simulink model "c28x_i2c_sensor"  (R2023b)
settings: Solver=FixedStepDiscrete  StartTime=0.0  StopTime=Inf  FixedStep=Auto  RelTol=1e-3  EnableMultiTasking=on
undefined symbols (not defined in the file): dataType
libraries: c280xlib x7, simulink x3, demo_controls x1, svdschedulerlib x1, svdutilitieslib x1
settings Model: SimulationMode=external  ExtModeTrigDuration=8  Creator=The MathWorks, Inc.  LastModifiedBy=13571
settings SolverCC: AlgebraicLoopSolver=TrustRegion  AutoInsertRateTranBlk=on
settings DataIOCC: LimitDataPoints=on  SaveFormat=Array  SaveOutput=off  SaveTime=off  ReturnWorkspaceOutputs=off
settings OptimizationCC: BlockReduction=off  ConditionallyExecuteInputs=off  DefaultParameterBehavior=Inlined  DefaultUnderspecifiedDataType=single  OptimizeBlockIOStorage=off  BufferReuse=off  GlobalBufferReuse=off  ExpressionFolding=off  ExpressionDepthLimit=2147483647  LocalBlockOutputs=off  InitFltsAndDblsToZero=on  LifeSpan=Inf  MaxStackSize=1024  EfficientTunableParamExpr=on
settings DebuggingCC: UnderspecifiedInitializationDetection=Classic  MergeDetectMultiDrivingBlocksExec=none  SolverPrmCheckMsg=warning  InheritedTsInSrcMsg=none  FcnCallInpInsideContextMsg=warning  UnconnectedInputMsg=warning  UnconnectedOutputMsg=warning  UnconnectedLineMsg=warning  AllowSymbolicDim=off  StateNameClashWarn=warning  SFUnexpectedBacktrackingDiag=warning  SFNoUnconditionalDefaultTransitionDiag=warning  SFExecutionAtInitializationDiag=none  ArithmeticOperatorsInVariantConditions=warning
settings HardwareCC: ProdBitPerChar=16  ProdBitPerInt=16  ProdBitPerPointer=32  ProdBitPerSizeT=32  ProdBitPerPtrDiffT=32  ProdLargestAtomicInteger=Integer  ProdLargestAtomicFloat=None  ProdWordSize=16  ProdLongLongMode=on  ProdHWDeviceType=Texas Instruments->C2000  TargetBitPerChar=16  TargetBitPerInt=16  TargetBitPerPointer=16  TargetIntDivRoundTo=Zero  TargetEndianess=LittleEndian  TargetWordSize=16  TargetHWDeviceType=TI C2000  HardwareBoardFeatureSet=SoCBlockset
settings ModelReferenceCC: EnableRefExpFcnMdlSchedulingChecks=on  ModelReferenceNumInstancesAllowed=Single  PropagateSignalLabelsOutOfModel=off
settings SFSimCC: SimUseLocalCustomCode=off  SimParseCustomCode=off  CustomCodeUndefinedFunction=UseInterfaceOnly
settings RTWCC: Description=Embedded Coder  SystemTargetFile=ert.tlc  HardwareBoard=TI Delfino F28379D LaunchPad  TemplateMakefile=ert_default_tmf  RTWUseLocalCustomCode=off  Toolchain=Texas Instruments Code Composer Studio (C2000)  CodeProfilingSaveOptions=MetricsOnly  DLArmComputeVersion=19.05
settings CodeAppCC: IgnoreCustomStorageClasses=off  CustomSymbolStrType=$N$R$M  StateflowObjectComments=on  InternalIdentifier=Classic
settings ERTTargetCC: CodeReplacementLibrary=TI C28x  MultiwordLength=2048  ExtModeTransport=5  ExtModeStaticAlloc=on  ExtModeAutomaticAllocSize=off  ExtModeStaticAllocSize=10000  ExtModeMexFile=ext_xcp  ExtModeIntrfLevel=Level2 - Open  ConvertIfToSwitch=off  SuppressUnreachableDefaultCases=off
settings ConfigComp: CovMetricSettings=dw  CovSaveCumulativeToWorkspaceVar=on  CovSaveSingleToWorkspaceVar=on  CovExternalEMLEnable=off  CovSFcnEnable=off

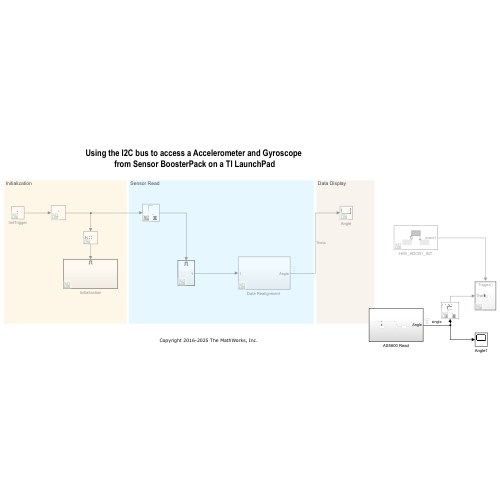
[thumbnail: Simulink's stored preview of the top-level diagram]
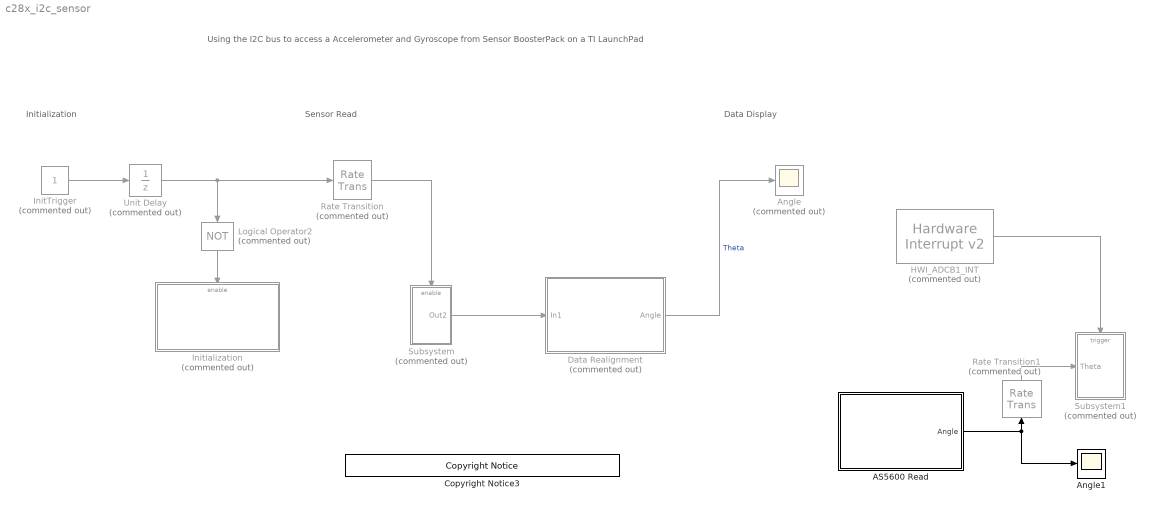
== system c28x_i2c_sensor ==
  note: Using the I2C bus to access a Accelerometer and Gyroscope
      | from Sensor BoosterPack on a TI LaunchPad
  note: Initialization
  note: Data Display
  note: Sensor Read
  AS5600 Read : Subsystem
  Angle : Scope  Commented=on
  Angle1 : Scope
  Copyright Notice3 : demo_controls/Copyright Notice  year=2016  prod=tic2000
  "Data Realignment " : Subsystem  Commented=on
  HWI_ADCB1_INT : svdschedulerlib/Hardware Interrupt v2  Commented=on  ISRGroup=ADC - Analog to Digital Converter  ISRName=ADCA1_INT  ISRNumber=32  NumEventsToServe=1  EventsList={'on','EOC event','1';'off','Overflow event','2';'off','Custom event','3'}  SelectedEvents={'event1'}  TaskPriority=30  DisablePreemption=off  ClearInterruptFlagsAtEndOfEvent=on  InterruptDefinitionFile=$(TARGET_ROOT)/registry/interrupts/F2837xS_interrupts.xml  HardwareBoard=F2837x  EnableSimPort=off
      settings: LibrarySourceBlock=c2000lib/Scheduling/Hardware Interrupt
  InitTrigger : Constant  Priority=10  Commented=on  OutDataTypeStr=uint16  SampleTime=15e-3
  Initialization : Subsystem  Commented=on
  Logical Operator2 : Logic  Commented=on  Operator=NOT  AllPortsSameDT=off  OutDataTypeStr=boolean
  Rate Transition : RateTransition  Commented=on  OutPortSampleTime=1e-3
  Rate Transition1 : RateTransition  Commented=on  Deterministic=off
  Subsystem : Subsystem  Commented=on
  Subsystem1 : Subsystem  Commented=on
  Unit Delay : UnitDelay  Commented=on  SampleTime=-1  HasFrameUpgradeWarning=on
  wires:
  Unit Delay/1 -> Rate Transition/1, Logical Operator2/1
  InitTrigger/1 -> Unit Delay/1
  "Data Realignment "/1(Angle) -> Angle/1  "Theta"
  Logical Operator2/1 -> Initialization/Enable
  Subsystem/1(Out2) -> "Data Realignment "/1(In1)
  Rate Transition/1 -> Subsystem/Enable
  HWI_ADCB1_INT/1 -> Subsystem1/Trigger
  AS5600 Read/1(Angle) -> Angle1/1, Rate Transition1/1
  Rate Transition1/1 -> Subsystem1/1(Theta)

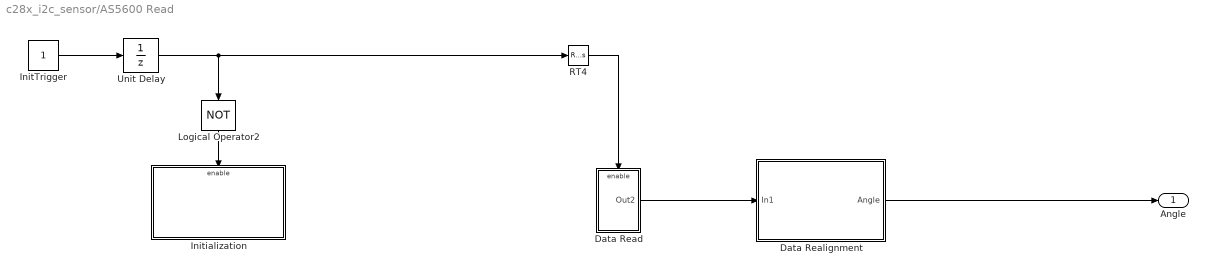
== system c28x_i2c_sensor/AS5600 Read ==
  Data Read : Subsystem
  "Data Realignment " : Subsystem
  InitTrigger : Constant  Priority=10  OutDataTypeStr=boolean  SampleTime=15e-3
  Initialization : Subsystem
  Logical Operator2 : Logic  Operator=NOT  AllPortsSameDT=off  OutDataTypeStr=boolean
  RT4 : RateTransition  Deterministic=off  OutPortSampleTime=1e-3
  Unit Delay : UnitDelay  SampleTime=-1  HasFrameUpgradeWarning=on
  Angle : Outport
  wires:
  InitTrigger/1 -> Unit Delay/1
  Logical Operator2/1 -> Initialization/Enable
  Unit Delay/1 -> RT4/1, Logical Operator2/1
  Data Read/1(Out2) -> "Data Realignment "/1(In1)
  RT4/1 -> Data Read/Enable
  "Data Realignment "/1(Angle) -> Angle/1

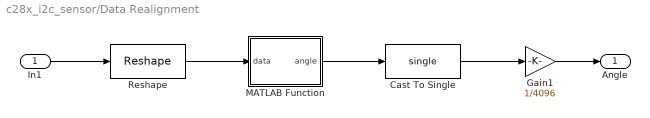
== system c28x_i2c_sensor/Data Realignment  ==
  In1 : Inport
  Cast To Single : DataTypeConversion  OutDataTypeStr=single  SaturateOnIntegerOverflow=off  RndMeth=Floor
  Gain1 : Gain  Gain=1/4096
  MATLAB Function : MATLAB Function  TreatAsAtomicUnit=on
  Reshape : Reshape  OutputDimensionality=Customize  OutputDimensions=[2,1]
  Angle : Outport  VectorParamsAs1DForOutWhenUnconnected=off
  wires:
  Reshape/1 -> MATLAB Function/1(data)
  In1/1 -> Reshape/1
  MATLAB Function/1(angle) -> Cast To Single/1
  Cast To Single/1 -> Gain1/1
  Gain1/1 -> Angle/1

== system c28x_i2c_sensor/Initialization ==
  Enable : EnablePort
  Address - Data read : Subsystem  TreatAsAtomicUnit=on
  Delay 1ms : Subsystem  TreatAsAtomicUnit=on
  Function-Call Generator : simulink/Ports & Subsystems/Function-Call Generator  sample_time=-1  numberOfIterations=1  DisallowWideOutput=off
  Function-Call Split1 : FunctionCallSplit  NumOutputPorts=2
  wires:
  Function-Call Generator/1 -> Function-Call Split1/1
  Function-Call Split1/1 -> Address - Data read/Trigger
  Function-Call Split1/2 -> Delay 1ms/Trigger

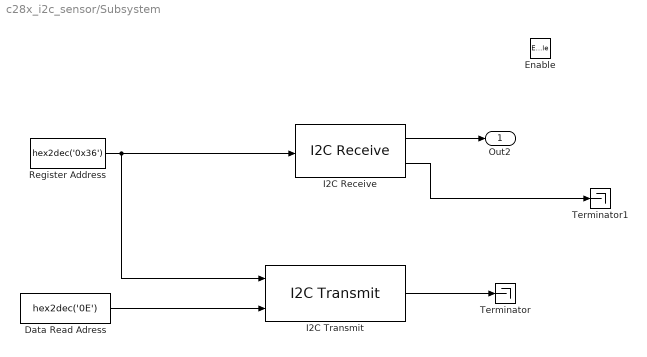
== system c28x_i2c_sensor/Subsystem ==
  Enable : EnablePort
  Data Read Adress : Constant  Priority=10  Value=hex2dec('0E')  OutDataTypeStr=uint8  SampleTime=-1
  I2C Receive : c280xlib/I2C Receive  Priority=10  selectModule=I2C_A  addrFormat=7-Bit addressing  saSource=Input port  SAR=54  bitCount=8  dataLength=2  initValue=0  NACK=off  STP=on  STR=on  sampleTime=-1  dataType=uint8
  I2C Transmit : c280xlib/I2C Transmit  Priority=20  selectModule=I2C_A  addrFormat=7-Bit addressing  saSource=Input port  SAR=0x36  bitCount=8  STP=off  RM=off  STR=on
  Register Address : Constant  Value=hex2dec('0x36')  OutDataTypeStr=uint8  SampleTime=-1
  Terminator : Terminator
  Terminator1 : Terminator
  Out2 : Outport  VectorParamsAs1DForOutWhenUnconnected=off
  wires:
  I2C Transmit/1 -> Terminator/1
  I2C Receive/1 -> Out2/1
  I2C Receive/2 -> Terminator1/1
  Data Read Adress/1 -> I2C Transmit/2
  Register Address/1 -> I2C Transmit/1, I2C Receive/1

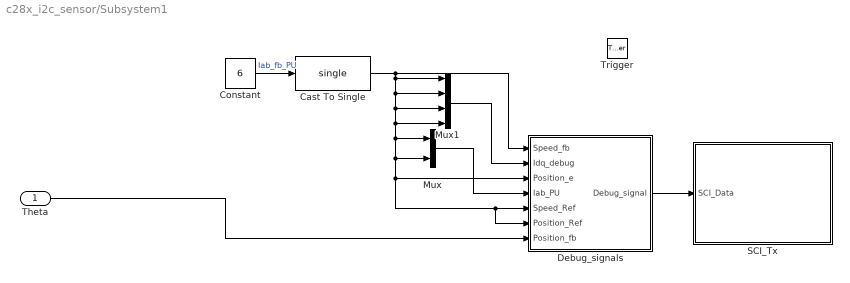
== system c28x_i2c_sensor/Subsystem1 ==
  Theta : Inport
  Trigger : TriggerPort  TriggerType=function-call  VariantControl=Variant  PortDimensions=1
  Cast To Single : DataTypeConversion  OutDataTypeStr=single  SaturateOnIntegerOverflow=off  RndMeth=Floor
  Constant : Constant  Value=6
  Debug_signals : Subsystem
  Mux : Mux  Inputs=2
  Mux1 : Mux
  SCI_Tx : Subsystem  Variant=on  VariantControlMode=sim codegen switching
  wires:
  Cast To Single/1 -> Mux1/3, Mux1/4, Mux/1, Mux/2, Debug_signals/3(Position_e), Debug_signals/6(Position_Ref), Debug_signals/5(Speed_Ref), Mux1/2, Mux1/1, Debug_signals/1(Speed_fb)
  Mux1/1 -> Debug_signals/2(Idq_debug)
  Constant/1 -> Cast To Single/1  "Iab_fb_PU"
  Debug_signals/1(Debug_signal) -> SCI_Tx/1(SCI_Data)
  Mux/1 -> Debug_signals/4(Iab_PU)
  Theta/1 -> Debug_signals/7(Position_fb)

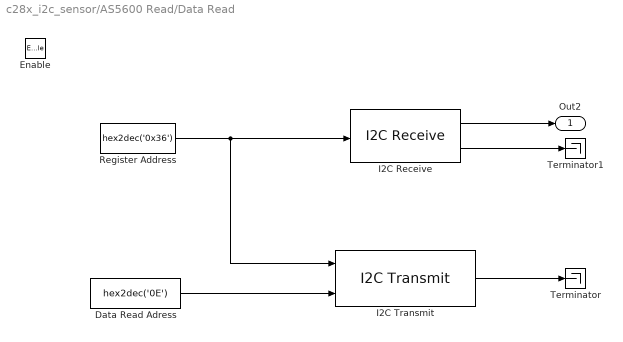
== system c28x_i2c_sensor/AS5600 Read/Data Read ==
  Enable : EnablePort
  Data Read Adress : Constant  Priority=10  Value=hex2dec('0E')  OutDataTypeStr=uint8  SampleTime=-1
  I2C Receive : c280xlib/I2C Receive  Priority=10  selectModule=I2C_A  addrFormat=7-Bit addressing  saSource=Input port  SAR=54  bitCount=8  dataLength=2  initValue=0  NACK=off  STP=on  STR=on  sampleTime=-1  dataType=uint8
  I2C Transmit : c280xlib/I2C Transmit  Priority=20  selectModule=I2C_A  addrFormat=7-Bit addressing  saSource=Input port  SAR=0x36  bitCount=8  STP=off  RM=off  STR=on
  Register Address : Constant  Value=hex2dec('0x36')  OutDataTypeStr=uint8  SampleTime=-1
  Terminator : Terminator
  Terminator1 : Terminator
  Out2 : Outport  VectorParamsAs1DForOutWhenUnconnected=off
  wires:
  I2C Transmit/1 -> Terminator/1
  I2C Receive/1 -> Out2/1
  I2C Receive/2 -> Terminator1/1
  Data Read Adress/1 -> I2C Transmit/2
  Register Address/1 -> I2C Transmit/1, I2C Receive/1

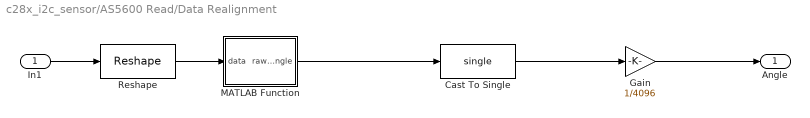
== system c28x_i2c_sensor/AS5600 Read/Data Realignment  ==
  In1 : Inport
  Cast To Single : DataTypeConversion  OutDataTypeStr=single  SaturateOnIntegerOverflow=off  RndMeth=Floor
  Gain : Gain  Gain=1/4096
  MATLAB Function : MATLAB Function  TreatAsAtomicUnit=on
  Reshape : Reshape  OutputDimensionality=Customize  OutputDimensions=[2,1]
  Angle : Outport  VectorParamsAs1DForOutWhenUnconnected=off
  wires:
  In1/1 -> Reshape/1
  Reshape/1 -> MATLAB Function/1(data)
  MATLAB Function/1(raw_angle) -> Cast To Single/1
  Cast To Single/1 -> Gain/1
  Gain/1 -> Angle/1

== system c28x_i2c_sensor/AS5600 Read/Initialization ==
  Enable : EnablePort
  Address - Data read : Subsystem  TreatAsAtomicUnit=on
  Delay 1ms : Subsystem  TreatAsAtomicUnit=on
  Function-Call Generator : simulink/Ports & Subsystems/Function-Call Generator  sample_time=-1  numberOfIterations=1  DisallowWideOutput=off
  Function-Call Split1 : FunctionCallSplit  NumOutputPorts=2
  wires:
  Function-Call Generator/1 -> Function-Call Split1/1
  Function-Call Split1/1 -> Address - Data read/Trigger
  Function-Call Split1/2 -> Delay 1ms/Trigger

== system c28x_i2c_sensor/Initialization/Address - Data read ==
  function : TriggerPort  TriggerType=function-call  VariantControl=Variant
  Data read address : Constant  Value=hex2dec('0x0E')  OutDataTypeStr=uint8  SampleTime=-1
  I2C Transmit1 : c280xlib/I2C Transmit  selectModule=I2C_A  addrFormat=7-Bit addressing  saSource=Input port  SAR=0x36  bitCount=8  STP=off  RM=off  STR=on
  Register Address : Constant  Value=hex2dec('0x36')  OutDataTypeStr=uint8  SampleTime=-1
  Terminator : Terminator
  wires:
  I2C Transmit1/1 -> Terminator/1
  Data read address/1 -> I2C Transmit1/2
  Register Address/1 -> I2C Transmit1/1

== system c28x_i2c_sensor/Initialization/Delay 1ms ==
  function : TriggerPort  TriggerType=function-call  VariantControl=Variant
  System Outputs : Subsystem  mask(System Outputs){ShowInLibBrowser=0}
      mask prompts: ShowInLibBrowser "Simulink:masks:CustCodeMaskParam1_MP"
      settings: CopyFcn=cccopyfcn(gcb)  OpenFcn=ccopenfcn('System Outputs Function')
      mask Help: eval('feval(''rtwprivate'',''rtwhelpview'',''rtw_sys_outputs_block'')');
      mask Display: disp('System\nOutputs');

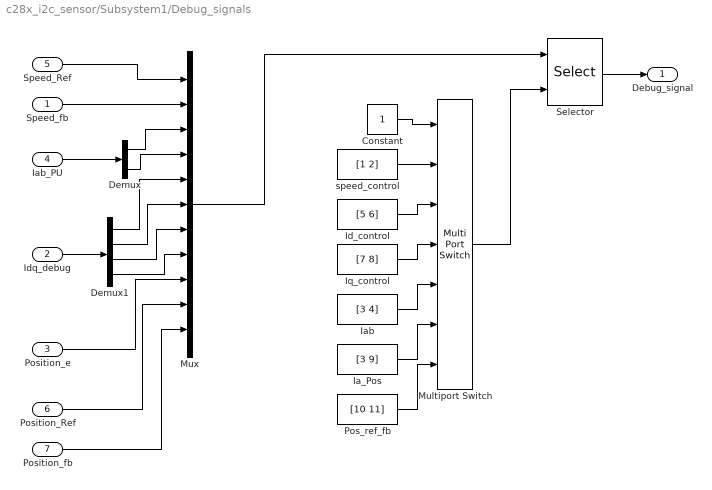
== system c28x_i2c_sensor/Subsystem1/Debug_signals ==
  Speed_fb : Inport
  Idq_debug : Inport  Port=2
  Position_e : Inport  Port=3
  Iab_PU : Inport  Port=4
  Speed_Ref : Inport  Port=5
  Position_Ref : Inport  Port=6
  Position_fb : Inport  Port=7
  Constant : Constant
  Demux : Demux  Outputs=2
  Demux1 : Demux
  Ia_Pos : Constant  Value=[3 9]  OutDataTypeStr=uint16  SampleTime=-1
  Iab : Constant  Value=[3 4]  OutDataTypeStr=uint16  SampleTime=-1
  Id_control : Constant  Value=[5 6]  OutDataTypeStr=uint16  SampleTime=-1
  Iq_control : Constant  Value=[7 8]  OutDataTypeStr=uint16  SampleTime=-1
  Multiport Switch : MultiPortSwitch  Inputs=6  DiagnosticForDefault=Warning  OutDataTypeStr=uint16  RndMeth=Simplest  SaturateOnIntegerOverflow=off  InputSameDT=off
  Mux : Mux  Inputs=11
  Pos_ref_fb : Constant  Value=[10 11]  OutDataTypeStr=uint16  SampleTime=-1
  Selector : Selector  InputPortWidth=11  IndexOptions=Index vector (port)  Indices=[1 3]  OutputSizes=1
  speed_control : Constant  Value=[1 2]  OutDataTypeStr=uint16  SampleTime=-1
  Debug_signal : Outport
  wires:
  speed_control/1 -> Multiport Switch/2
  Id_control/1 -> Multiport Switch/3
  Iq_control/1 -> Multiport Switch/4
  Iab/1 -> Multiport Switch/5
  Ia_Pos/1 -> Multiport Switch/6
  Multiport Switch/1 -> Selector/2
  Constant/1 -> Multiport Switch/1
  Selector/1 -> Debug_signal/1
  Iab_PU/1 -> Demux/1
  Demux/1 -> Mux/3
  Demux/2 -> Mux/4
  Demux1/1 -> Mux/5
  Demux1/2 -> Mux/6
  Demux1/3 -> Mux/7
  Demux1/4 -> Mux/8
  Idq_debug/1 -> Demux1/1
  Mux/1 -> Selector/1
  Position_e/1 -> Mux/9
  Speed_Ref/1 -> Mux/1
  Speed_fb/1 -> Mux/2
  Pos_ref_fb/1 -> Multiport Switch/7
  Position_Ref/1 -> Mux/10
  Position_fb/1 -> Mux/11

== system c28x_i2c_sensor/Subsystem1/SCI_Tx ==
  SCI_Data : Inport
  Code Generation : Subsystem  VariantControl=(codegen)
  Simulation : Subsystem  VariantControl=(sim)

== system c28x_i2c_sensor/AS5600 Read/Initialization/Address - Data read ==
  function : TriggerPort  TriggerType=function-call  VariantControl=Variant
  Data read address : Constant  Value=hex2dec('0x0E')  OutDataTypeStr=uint8  SampleTime=-1
  I2C Transmit1 : c280xlib/I2C Transmit  selectModule=I2C_A  addrFormat=7-Bit addressing  saSource=Input port  SAR=0x36  bitCount=8  STP=off  RM=off  STR=on
  Register Address : Constant  Value=hex2dec('0x36')  OutDataTypeStr=uint8  SampleTime=-1
  Terminator : Terminator
  wires:
  I2C Transmit1/1 -> Terminator/1
  Data read address/1 -> I2C Transmit1/2
  Register Address/1 -> I2C Transmit1/1

== system c28x_i2c_sensor/AS5600 Read/Initialization/Delay 1ms ==
  function : TriggerPort  TriggerType=function-call  VariantControl=Variant
  System Outputs : Subsystem  mask(System Outputs){ShowInLibBrowser=0}
      mask prompts: ShowInLibBrowser "Simulink:masks:CustCodeMaskParam1_MP"
      settings: CopyFcn=cccopyfcn(gcb)  OpenFcn=ccopenfcn('System Outputs Function')
      mask Help: eval('feval(''rtwprivate'',''rtwhelpview'',''rtw_sys_outputs_block'')');
      mask Display: disp('System\nOutputs');

== system c28x_i2c_sensor/Initialization/Delay 1ms/System Outputs ==

== system c28x_i2c_sensor/Subsystem1/SCI_Tx/Code Generation ==
  SCI_Data : Inport
  Data_Conditioning_Tx : Subsystem  Variant=on
  Data_Logging : Subsystem
  Demux2 : Demux  Outputs=2
  While Iterator Subsystem : Subsystem  TreatAsAtomicUnit=on
  wires:
  Demux2/2 -> While Iterator Subsystem/2(Iteration)  "SCI_Tx_Iteration"
  Demux2/1 -> While Iterator Subsystem/1(Data)  "SCI_Tx_Data"
  SCI_Data/1 -> Data_Conditioning_Tx/1(In1)
  Data_Logging/1(SCI_Tx) -> Demux2/1
  Data_Conditioning_Tx/1(Data_Log) -> Data_Logging/1(Data_Log)

== system c28x_i2c_sensor/Subsystem1/SCI_Tx/Simulation ==
  SCI_Data : Inport
  Demux : Demux  Outputs=2
  Terminator1 : Terminator
  Terminator2 : Terminator
  wires:
  SCI_Data/1 -> Demux/1
  Demux/1 -> Terminator1/1
  Demux/2 -> Terminator2/1

== system c28x_i2c_sensor/AS5600 Read/Initialization/Delay 1ms/System Outputs ==

== system c28x_i2c_sensor/Subsystem1/SCI_Tx/Code Generation/Data_Conditioning_Tx ==
  In1 : Inport
  Data_Type_Fixed_Point : Subsystem  VariantControl=~isequal(dataType,'single')
  Data_Type_Float : Subsystem  VariantControl=isequal(dataType, 'single')
  Data_Log : Outport

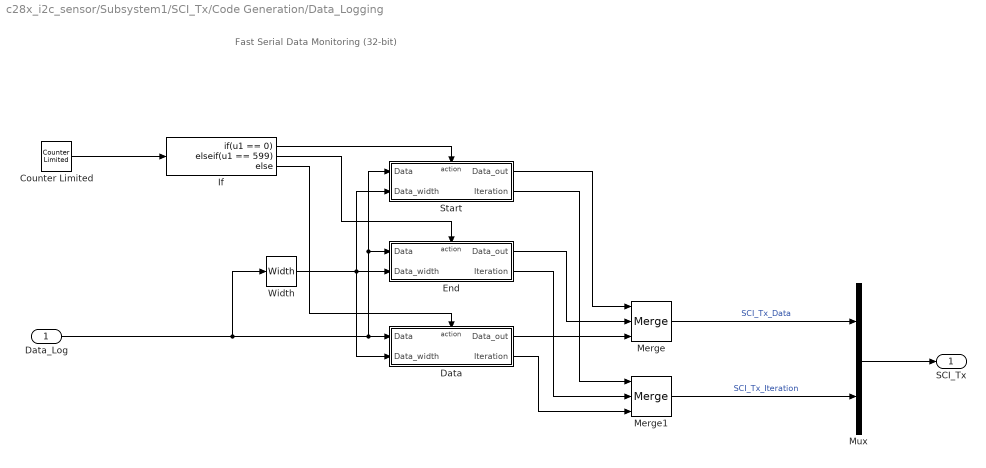
== system c28x_i2c_sensor/Subsystem1/SCI_Tx/Code Generation/Data_Logging ==
  note: Fast Serial Data Monitoring (32-bit)
  Data_Log : Inport
  Counter Limited : simulink/Sources/Counter Limited  uplimit=600-1  tsamp=-1
  Data : Subsystem  TreatAsAtomicUnit=on
  End : Subsystem  TreatAsAtomicUnit=on
  If : If  IfExpression=u1 == 0  ElseIfExpressions=u1 == 599
  Merge : Merge  Inputs=3
  Merge1 : Merge  Inputs=3
  Mux : Mux  Inputs=2
  Start : Subsystem  TreatAsAtomicUnit=on
  Width : Width  OutDataTypeMode=All ports same datatype  DataType=uint16
  SCI_Tx : Outport
  wires:
  If/3 -> Data/Action
  Data/1(Data_out) -> Merge/3
  Width/1 -> Data/2(Data_width), Start/2(Data_width), End/2(Data_width)
  Merge/1 -> Mux/1  "SCI_Tx_Data"
  Counter Limited/1 -> If/1
  Start/2(Iteration) -> Merge1/1
  Start/1(Data_out) -> Merge/1
  If/2 -> End/Action
  Merge1/1 -> Mux/2  "SCI_Tx_Iteration"
  If/1 -> Start/Action
  End/1(Data_out) -> Merge/2
  End/2(Iteration) -> Merge1/2
  Data/2(Iteration) -> Merge1/3
  Mux/1 -> SCI_Tx/1
  Data_Log/1 -> Width/1, Start/1(Data), End/1(Data), Data/1(Data)

== system c28x_i2c_sensor/Subsystem1/SCI_Tx/Code Generation/While Iterator Subsystem ==
  Data : Inport
  Iteration : Inport  Port=2
  Add : Sum  Inputs=+-  OutDataTypeStr=Inherit: Same as first input
  Index Vector : MultiPortSwitch  Inputs=1  SaturateOnIntegerOverflow=off  InputSameDT=off
  SCI Transmit : c280xlib/SCI Transmit  sciModule=A  dataHead=''  dataTail=''  frameSize=1  blockingMode=on  outputStatus=off
  While Iterator : WhileIterator  MaxIters=-1  WhileBlockType=do-while  ShowIterationPort=on  OutputDataType=int16
  wires:
  While Iterator/1 -> Add/2, Index Vector/1
  Data/1 -> Index Vector/2
  Index Vector/1 -> SCI Transmit/1
  Add/1 -> While Iterator/1
  Iteration/1 -> Add/1

== system c28x_i2c_sensor/Subsystem1/SCI_Tx/Code Generation/Data_Conditioning_Tx/Data_Type_Fixed_Point ==
  In1 : Inport
  Data Type Conversion : DataTypeConversion  OutDataTypeStr=fixdt(1,32,28)  RndMeth=Simplest  SaturateOnIntegerOverflow=off
  Data Type Conversion3 : DataTypeConversion  OutDataTypeStr=uint32  ConvertRealWorld=Stored Integer (SI)  RndMeth=Simplest  SaturateOnIntegerOverflow=off
  Data_Log : Outport
  wires:
  In1/1 -> Data Type Conversion/1
  Data Type Conversion3/1 -> Data_Log/1
  Data Type Conversion/1 -> Data Type Conversion3/1

== system c28x_i2c_sensor/Subsystem1/SCI_Tx/Code Generation/Data_Conditioning_Tx/Data_Type_Float ==
  In1 : Inport
  Byte Pack : svdutilitieslib/Byte Pack  maskPackedDataType=uint32  datatypes={'single'}  byteAlign=4  blockPlatform=tic2000
  Data_Log : Outport
  wires:
  Byte Pack/1 -> Data_Log/1
  In1/1 -> Byte Pack/1

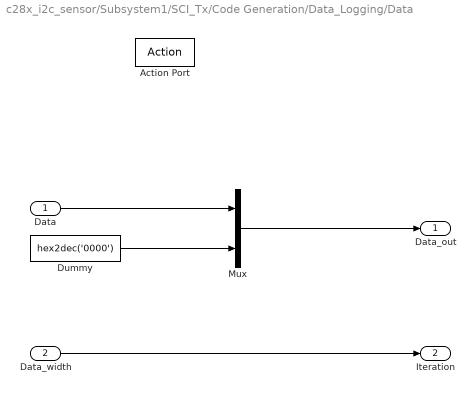
== system c28x_i2c_sensor/Subsystem1/SCI_Tx/Code Generation/Data_Logging/Data ==
  Data : Inport
  Data_width : Inport  Port=2
  Action Port : ActionPort  ActionPortLabel=else
  Dummy : Constant  Value=hex2dec('0000')  OutDataTypeStr=uint32
  Mux : Mux  Inputs=2
  Data_out : Outport  VectorParamsAs1DForOutWhenUnconnected=off
  Iteration : Outport  Port=2  VectorParamsAs1DForOutWhenUnconnected=off
  wires:
  Data_width/1 -> Iteration/1
  Data/1 -> Mux/1
  Dummy/1 -> Mux/2
  Mux/1 -> Data_out/1

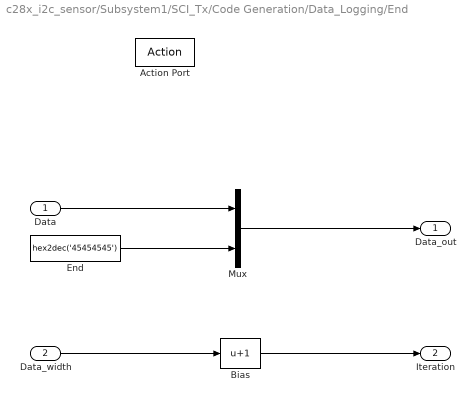
== system c28x_i2c_sensor/Subsystem1/SCI_Tx/Code Generation/Data_Logging/End ==
  Data : Inport
  Data_width : Inport  Port=2
  Action Port : ActionPort  ActionPortLabel=elseif(u1 == 599)
  Bias : Bias  Bias=1  SaturateOnIntegerOverflow=off
  End : Constant  Value=hex2dec('45454545')  OutDataTypeStr=uint32
  Mux : Mux  Inputs=2
  Data_out : Outport  VectorParamsAs1DForOutWhenUnconnected=off
  Iteration : Outport  Port=2  VectorParamsAs1DForOutWhenUnconnected=off
  wires:
  Data/1 -> Mux/1
  Data_width/1 -> Bias/1
  Bias/1 -> Iteration/1
  End/1 -> Mux/2
  Mux/1 -> Data_out/1

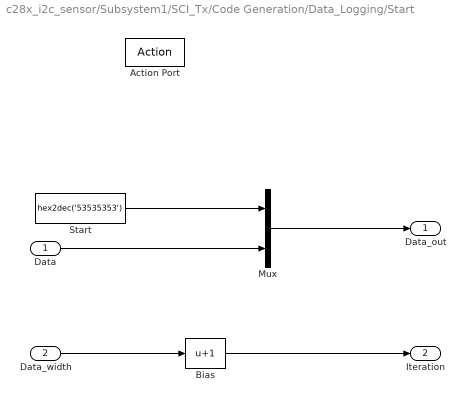
== system c28x_i2c_sensor/Subsystem1/SCI_Tx/Code Generation/Data_Logging/Start ==
  Data : Inport
  Data_width : Inport  Port=2
  Action Port : ActionPort  ActionPortLabel=if(u1 == 0)
  Bias : Bias  Bias=1  SaturateOnIntegerOverflow=off
  Mux : Mux  Inputs=2
  Start : Constant  Value=hex2dec('53535353')  OutDataTypeStr=uint32
  Data_out : Outport  VectorParamsAs1DForOutWhenUnconnected=off
  Iteration : Outport  Port=2  VectorParamsAs1DForOutWhenUnconnected=off
  wires:
  Data/1 -> Mux/2
  Data_width/1 -> Bias/1
  Bias/1 -> Iteration/1
  Start/1 -> Mux/1
  Mux/1 -> Data_out/1

== matlab function c28x_i2c_sensor/AS5600 Read/Data Realignment /MATLAB Function ==
  data: data input; raw_angle output
function raw_angle = fcn(data)
    %#codegen
    
    % 提取 MSB 和 LSB
    msb = data(1);
    lsb = data(2);
    
    % 合并 MSB 和 LSB 到一个 16-bit 整数
    raw_angle = bitshift(uint16(msb), 8) + uint16(lsb);
    
end

== matlab function c28x_i2c_sensor/Data Realignment /MATLAB Function ==
  data: data input; angle output
function angle = fcn(data)
    %#codegen
    
    % 提取 MSB 和 LSB
    msb = data(1);
    lsb = data(2);
    
    % 合并 MSB 和 LSB 到一个 16-bit 整数
    raw_angle = bitshift(uint16(msb), 8) + uint16(lsb);
    
    % 转换为角度 (假设 AS5600 输出范围是 0~4095 对应 0°~360°)
    angle = raw_angle; %double(raw_angle) * 360 / 4096; %
end
